simulink model "lab2"  (R2021b)
settings: Solver=VariableStepAuto  StartTime=0.0  StopTime=10  RelTol=1e-3
settings Model: Creator=Venik  LastModifiedBy=Venik

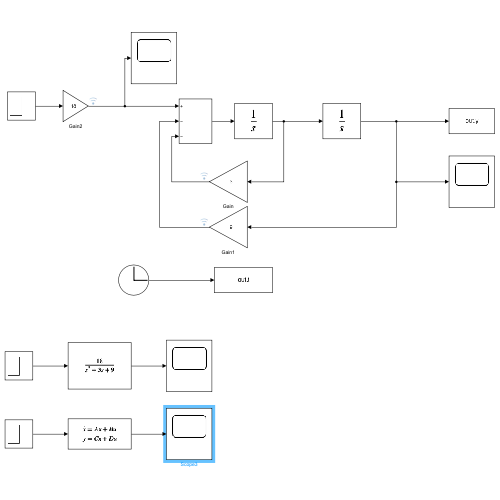
[thumbnail: Simulink's stored preview of the top-level diagram]
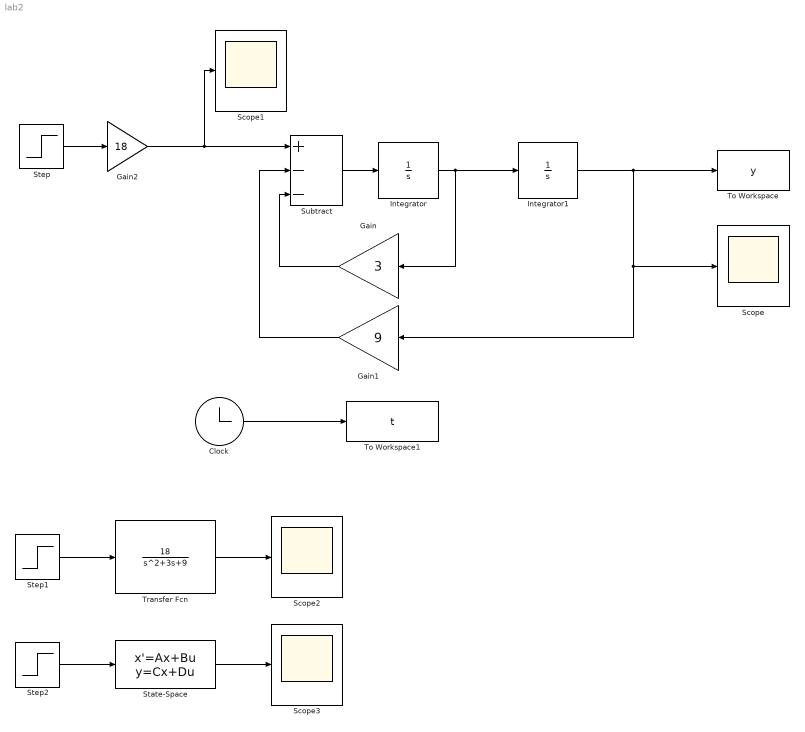
== system lab2 ==
  Clock : Clock
  Gain : Gain  Gain=3
  Gain1 : Gain  Gain=9
  Gain2 : Gain  Gain=18
  Integrator : Integrator
  Integrator1 : Integrator
  Scope{,1..3} (4 alike) : Scope
  State-Space : StateSpace  A=[-3 -9; 1 0]  B=[1;0]  C=[0 18]  D=0  InitialCondition=0
  Step : Step  SampleTime=0
  Step1 : Step  SampleTime=0
  Step2 : Step  SampleTime=0
  Subtract : Sum  Inputs=+--
  To Workspace : ToWorkspace  VariableName=y  SaveFormat=Timeseries  SampleTime=-1
  To Workspace1 : ToWorkspace  VariableName=t  SampleTime=-1
  Transfer Fcn : TransferFcn  Numerator=[18]  Denominator=[1 3 9]
  wires:
  Clock/1 -> To Workspace1/1
  Subtract/1 -> Integrator/1
  Integrator/1 -> Gain/1, Integrator1/1
  Gain/1 -> Subtract/3
  Integrator1/1 -> Scope/1, Gain1/1, To Workspace/1
  Step/1 -> Gain2/1
  Gain2/1 -> Scope1/1, Subtract/1
  Gain1/1 -> Subtract/2
  Step1/1 -> Transfer Fcn/1
  Transfer Fcn/1 -> Scope2/1
  Step2/1 -> State-Space/1
  State-Space/1 -> Scope3/1
